simulink model "DC_motor"  (R2022b)
settings: Solver=VariableStepAuto  StartTime=0.0  StopTime=10.0  RelTol=1e-3
InitFcn:
  | R = 1;
  | L = 0.5;
  | K = 0.01;
  | b = 0.1;
  | J = 0.01;
  | Kt = 0.01;
  | 
  | A = [-R/L -K/L; Kt/J -b/J];
  | B = [1/L; 0];
  | C = [0 1];
  | D = 0;
  | 
  | [Num Den] = ss2tf(A,B,C,D);
  | G = tf(Num, Den);
undefined symbols (not defined in the file or in its folder): Den, Num
settings Model: Creator=user  LastModifiedBy=user

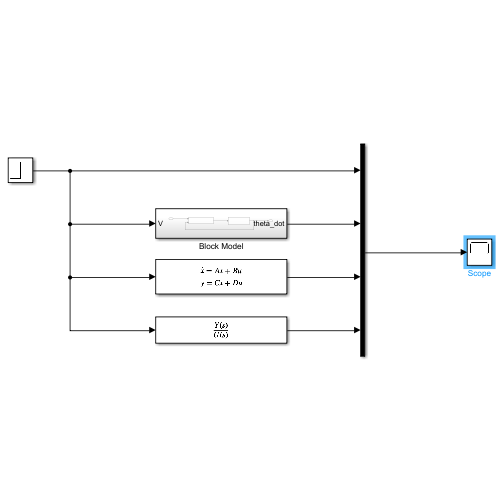
[thumbnail: Simulink's stored preview of the top-level diagram]
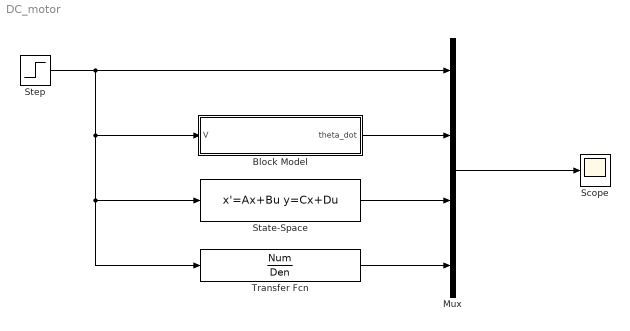
== system DC_motor ==
  Block Model : Subsystem
  Mux : Mux
  Scope : Scope
  State-Space : StateSpace  A=A  B=B  C=C  D=D  InitialCondition=0
  Step : Step  After=10  SampleTime=0
  Transfer Fcn : TransferFcn  Numerator=Num  Denominator=Den
  wires:
  Step/1 -> Block Model/1(V), Transfer Fcn/1, State-Space/1, Mux/1
  Mux/1 -> Scope/1
  Block Model/1(theta_dot) -> Mux/2
  State-Space/1 -> Mux/3
  Transfer Fcn/1 -> Mux/4

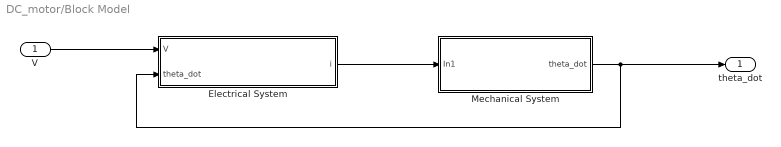
== system DC_motor/Block Model ==
  V : Inport
  Electrical System : Subsystem
  Mechanical System : Subsystem
  theta_dot : Outport
  wires:
  Mechanical System/1(theta_dot) -> theta_dot/1, Electrical System/2(theta_dot)
  V/1 -> Electrical System/1(V)
  Electrical System/1(i) -> Mechanical System/1(In1)

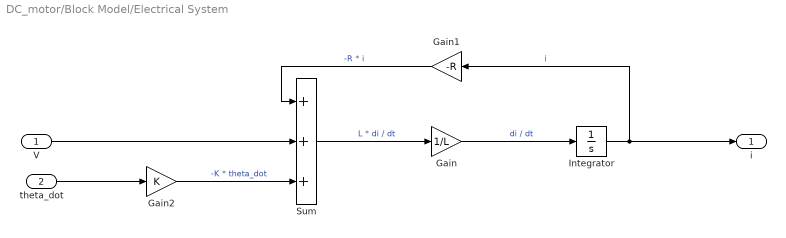
== system DC_motor/Block Model/Electrical System ==
  V : Inport
  theta_dot : Inport  Port=2
  Gain : Gain  Gain=1/L
  Gain1 : Gain  Gain=-R
  Gain2 : Gain  Gain=K
  Integrator : Integrator
  Sum : Sum  Inputs=+++
  i : Outport
  wires:
  Gain1/1 -> Sum/1  "-R * i"
  Gain/1 -> Integrator/1  "di / dt"
  theta_dot/1 -> Gain2/1
  Gain2/1 -> Sum/3  "-K * theta_dot"
  Integrator/1 -> i/1, Gain1/1  "i"
  Sum/1 -> Gain/1  "L * di / dt"
  V/1 -> Sum/2

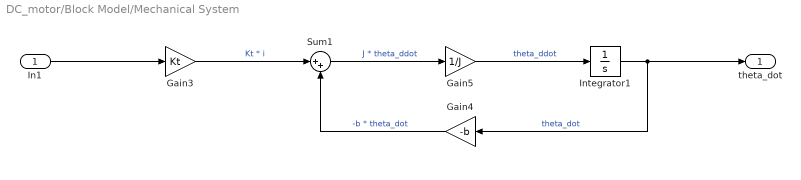
== system DC_motor/Block Model/Mechanical System ==
  In1 : Inport
  Gain3 : Gain  Gain=Kt
  Gain4 : Gain  Gain=-b
  Gain5 : Gain  Gain=1/J
  Integrator1 : Integrator
  Sum1 : Sum  Inputs=|++
  theta_dot : Outport
  wires:
  In1/1 -> Gain3/1
  Gain5/1 -> Integrator1/1  "theta_ddot"
  Integrator1/1 -> theta_dot/1, Gain4/1  "theta_dot"
  Sum1/1 -> Gain5/1  "J * theta_ddot"
  Gain3/1 -> Sum1/1  "Kt * i"
  Gain4/1 -> Sum1/2  "-b * theta_dot"
